simulink model "ACC_Decision_SPPVT_Simple"  (R2024b)
settings: Solver=FixedStepAuto  StartTime=0.0  StopTime=10.0  FixedStep=0.05  RelTol=1e-3
settings Model: Creator=ZhaoY  LastModifiedBy=ZhaoY

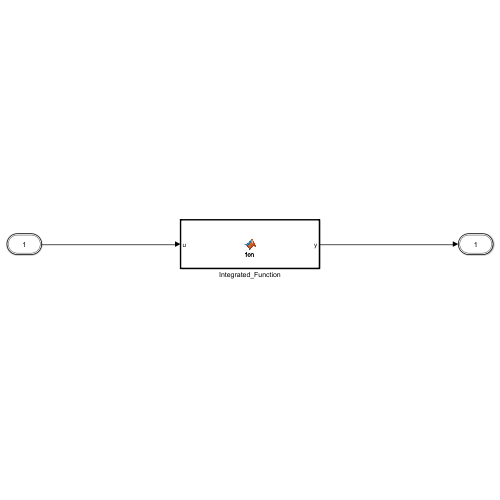
[thumbnail: Simulink's stored preview of the top-level diagram]
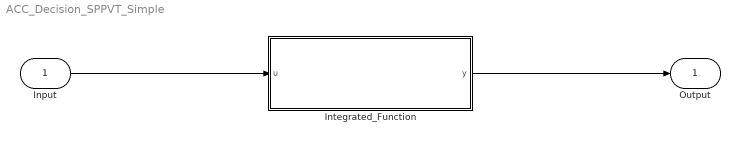
== system ACC_Decision_SPPVT_Simple ==
  Input : Inport  OutDataTypeStr=Bus: DecisionSPPVTInput
  Integrated_Function : MATLAB Function  TreatAsAtomicUnit=on
  Output : Outport  OutDataTypeStr=Bus: DecisionSPPVTOutput
  wires:
  Input/1 -> Integrated_Function/1(u)
  Integrated_Function/1(y) -> Output/1

== matlab function ACC_Decision_SPPVT_Simple/Integrated_Function ==
  data: u input; y output
function y = fcn(u)

y = u;
